simulink model "H250Model2019b"  (R2019b)
settings: Solver=ode4  StartTime=0.0  StopTime=inf  FixedStep=Ts  RelTol=1e-3
values from neighbouring files (symbols this model uses):
  ModelFail_env_P_wind = [0 0 0]    [F450DegradedParamInit.m]    (also in H250DegradedParamInit.m; H250ModelParam4S.m; H333DegradedParamInit4S.m)
  ModelFail_motor_isEnable = 0    [F450DegradedParamInit.m]    (also in H250DegradedParamInit.m; H250ModelParam4S.m; H333DegradedParamInit4S.m)
  ModelFail_motor_kCt = [1 1 1 1 1 1 1 1]    [F450DegradedParamInit.m]    (also in H250DegradedParamInit.m; H250ModelParam4S.m; H333DegradedParamInit4S.m)
  ModelFail_motor_kTc = [1 1 1 1 1 1 1 1]    [F450DegradedParamInit.m]    (also in H250DegradedParamInit.m; H250ModelParam4S.m; H333DegradedParamInit4S.m)
  ModelFail_motor_kw = [1 1 1 1 1 1 1 1]    [F450DegradedParamInit.m]    (also in H250DegradedParamInit.m; H250ModelParam4S.m; H333DegradedParamInit4S.m)
  ModelInit_motorInitRate = 0    [F450DegradedParamInit.m]    (also in H250DegradedParamInit.m; H250ModelParam4S.m; H333DegradedParamInit4S.m)
  ModelParam_Airframe_CMP = [0 0 0]    [F450DegradedParamInit.m]    (also in H250DegradedParamInit.m; H250ModelParam4S.m; H333DegradedParamInit4S.m)
  ModelParam_Airframe_J = [0.0194 0 0;0 0.0194 0;0 0 0.0291]    [F450DegradedParamInit.m]    (also in H250DegradedParamInit.m = [0.0056 0 0;0 0.0056 0;0 0 0.0104]; H250ModelParam4S.m = [0.0056 0 0;0 0.0056 0;0 0 0.0104]; H333DegradedParamInit4S.m = [0.012 0 0;0 0.012 0;0 0 0.02])
  ModelParam_Airframe_m = 1.31    [F450DegradedParamInit.m]    (also in H250DegradedParamInit.m = 0.752; H250ModelParam4S.m = 0.752; H333DegradedParamInit4S.m = 1.13)
  ModelParam_envAltitude = 0    [F450DegradedParamInit.m]    (also in H250DegradedParamInit.m; H250ModelParam4S.m; H333DegradedParamInit4S.m)
  ModelParam_envC_d = 0.055    [F450DegradedParamInit.m]    (also in H250DegradedParamInit.m; H250ModelParam4S.m; H333DegradedParamInit4S.m)
  ModelParam_envC_md = [0.001 0.001 0.00058]    [F450DegradedParamInit.m]    (also in H250DegradedParamInit.m = [0.001 0.001 0.00040]; H250ModelParam4S.m = [0.001 0.001 0.00040]; H333DegradedParamInit4S.m = [0.001 0.001 0.0002])
  ModelParam_GPSEphFinal = 0.3    [F450DegradedParamInit.m]    (also in H250DegradedParamInit.m; H250ModelParam4S.m; H333DegradedParamInit4S.m)
  ModelParam_GPSEpvFinal = 0.4    [F450DegradedParamInit.m]    (also in H250DegradedParamInit.m; H250ModelParam4S.m; H333DegradedParamInit4S.m)
  ModelParam_GPSFix3DFix = 3    [F450DegradedParamInit.m]    (also in H250DegradedParamInit.m; H250ModelParam4S.m; H333DegradedParamInit4S.m)
  ModelParam_GPSSatsVisible = 10    [F450DegradedParamInit.m]    (also in H250DegradedParamInit.m; H250ModelParam4S.m; H333DegradedParamInit4S.m)
  ModelParam_motorCr = 842.1    [F450DegradedParamInit.m]    (also in H250DegradedParamInit.m = 0; H250ModelParam4S.m = 0; H333DegradedParamInit4S.m = 0)
  ModelParam_motorFitType = 1    [F450DegradedParamInit.m]    (also in H250DegradedParamInit.m = 2; H250ModelParam4S.m = 2; H333DegradedParamInit4S.m = 2)
  ModelParam_motorJm = 0.0000687    (= 6.87e-05)    [F450DegradedParamInit.m]    (also in H250DegradedParamInit.m = 8.8493e-06; H250ModelParam4S.m = 8.8493e-06; H333DegradedParamInit4S.m = 8.8493e-06)
  ModelParam_motorMinThr = 0.05    [F450DegradedParamInit.m]    (also in H250DegradedParamInit.m = 0.148; H250ModelParam4S.m = 0.148; H333DegradedParamInit4S.m = 0.11)
  ModelParam_motorRateCurveCoeffi = [0 0 0]    [F450DegradedParamInit.m]    (also in H250DegradedParamInit.m = [-1364 3870 -372.4]; H250ModelParam4S.m = [-2143 5113 -458.4]; H333DegradedParamInit4S.m = [-1057 2662 -94.98])
  ModelParam_motorTc = 0.0214    [F450DegradedParamInit.m]    (also in H250DegradedParamInit.m = 0.035; H250ModelParam4S.m = 0.032; H333DegradedParamInit4S.m = 0.035)
  ModelParam_motorWb = 0    [F450DegradedParamInit.m]    (also in H250DegradedParamInit.m; H250ModelParam4S.m; H333DegradedParamInit4S.m)
  ModelParam_NoiseVarAcc0 = [0.1 0.1 0.1]    [F450DegradedParamInit.m]    (also in H250DegradedParamInit.m; H250ModelParam4S.m = [0.01 0.01 0.01]; H333DegradedParamInit4S.m)
  ModelParam_NoiseVarAcc1 = [0.1 0.1 0.1]    [F450DegradedParamInit.m]    (also in H250DegradedParamInit.m; H250ModelParam4S.m = [0.01 0.01 0.01]; H333DegradedParamInit4S.m)
  ModelParam_NoiseVarGPS_P0 = [1e-5 1e-5 1e-5]    [F450DegradedParamInit.m]    (also in H250DegradedParamInit.m; H250ModelParam4S.m; H333DegradedParamInit4S.m)
  ModelParam_NoiseVarGPS_V0 = [1e-5 1e-5 1e-5]    [F450DegradedParamInit.m]    (also in H250DegradedParamInit.m; H250ModelParam4S.m; H333DegradedParamInit4S.m)
  ModelParam_NoiseVarGyro0 = [0.0005 0.0005 0.0005]    [F450DegradedParamInit.m]    (also in H250DegradedParamInit.m; H250ModelParam4S.m; H333DegradedParamInit4S.m)
  ModelParam_NoiseVarGyro1 = [0.004 0.004 0.004]    [F450DegradedParamInit.m]    (also in H250DegradedParamInit.m; H250ModelParam4S.m; H333DegradedParamInit4S.m)
  ModelParam_NoiseVarMag0 = [0.000002 0.000002 0.000002]    [F450DegradedParamInit.m]    (also in H250DegradedParamInit.m; H250ModelParam4S.m; H333DegradedParamInit4S.m)
  ModelParam_NoiseVarMag1 = [0.0001 0.0001 0.0001]    [F450DegradedParamInit.m]    (also in H250DegradedParamInit.m; H250ModelParam4S.m; H333DegradedParamInit4S.m)
  ModelParam_PositionAcc0 = [0.071  0  -0.1365]    [F450DegradedParamInit.m]    (also in H250DegradedParamInit.m; H250ModelParam4S.m; H333DegradedParamInit4S.m)
  ModelParam_PositionAcc1 = [0.071  0  -0.1365]    [F450DegradedParamInit.m]    (also in H250DegradedParamInit.m; H250ModelParam4S.m; H333DegradedParamInit4S.m)
  ModelParam_rotorCt = 1.681e-05    [F450DegradedParamInit.m]    (also in H250DegradedParamInit.m = 1.448e-06; H250ModelParam4S.m = 1.345e-06; H333DegradedParamInit4S.m = 7.586e-06)
  ModelParam_WalkNoiseVarAcc0 = [0.001 0.001 0.001]    [F450DegradedParamInit.m]    (also in H250DegradedParamInit.m; H250ModelParam4S.m; H333DegradedParamInit4S.m)
  ModelParam_WalkNoiseVarAcc1 = [0.001 0.001 0.001]    [F450DegradedParamInit.m]    (also in H250DegradedParamInit.m; H250ModelParam4S.m; H333DegradedParamInit4S.m)
  ModelParam_WalkNoiseVarGPS_P0 = [0.01 0.01 0.01]    [F450DegradedParamInit.m]    (also in H250DegradedParamInit.m; H250ModelParam4S.m = [0 0 0]; H333DegradedParamInit4S.m)
  ModelParam_WalkNoiseVarGPS_V0 = [0.01 0.01 0.01]    [F450DegradedParamInit.m]    (also in H250DegradedParamInit.m; H250ModelParam4S.m = [0 0 0]; H333DegradedParamInit4S.m)
  ModelParam_WalkNoiseVarGyro0 = [0.00004 0.00004 0.00004]    [F450DegradedParamInit.m]    (also in H250DegradedParamInit.m; H250ModelParam4S.m; H333DegradedParamInit4S.m)
  ModelParam_WalkNoiseVarGyro1 = [0.00004 0.00004 0.00004]    [F450DegradedParamInit.m]    (also in H250DegradedParamInit.m; H250ModelParam4S.m; H333DegradedParamInit4S.m)
  ModelParam_WalkNoiseVarMag0 = [0.000001 0.000001 0.000001]    [F450DegradedParamInit.m]    (also in H250DegradedParamInit.m; H250ModelParam4S.m; H333DegradedParamInit4S.m)
  ModelParam_WalkNoiseVarMag1 = [0.000001 0.000001 0.000001]    [F450DegradedParamInit.m]    (also in H250DegradedParamInit.m; H250ModelParam4S.m; H333DegradedParamInit4S.m)
  MulticopterLayoutConfig = 1    [F450DegradedParamInit.m]    (also in H250DegradedParamInit.m = 6; H250ModelParam4S.m = 7; H333DegradedParamInit4S.m = 8)
  RflySimDisplayUAVType = 3    [F450DegradedParamInit.m]    (also in H250DegradedParamInit.m; H250ModelParam4S.m; H333DegradedParamInit4S.m)
  Ts = 1/1000    (= 0.001)    [F450DegradedParamInit.m]    (also in H250DegradedParamInit.m; H250ModelParam4S.m; H333DegradedParamInit4S.m)
undefined symbols (not defined in the file or in its folder): Earth, WGS84
libraries: aerolibnav x5, aerolibtransform2 x3, sharedtransform x3, aerolibutil x2, sharedutil x1, shared6dof x1, aerolibasang x1, aerolibatmos2 x1, aerolibconvert2 x1
(part 1 of 3)
settings Model: Creator=Jinrui  LastModifiedBy=kcx06
settings OptimizationCC: EfficientTunableParamExpr=on
settings DebuggingCC: ParameterTunabilityLossMsg=error  ArithmeticOperatorsInVariantConditions=warning
settings SFSimCC: SimUseLocalCustomCode=off  MATLABDynamicMemAlloc=off  CustomCodeUndefinedFunction=UseInterfaceOnly
settings RTWCC: SystemTargetFile=ert.tlc  GenCodeOnly=on  GenerateMakefile=off  PackageGeneratedCodeAndArtifacts=on  PackageName=MulticopterModel  TemplateMakefile=ert_default_tmf  RTWUseLocalCustomCode=off  TargetLang=C++  RTWCompilerOptimization=on
settings CodeAppCC: ForceParamTrailComments=on  OperatorAnnotations=on  SimulinkDataObjDesc=on  SFDataObjDesc=on  MATLABFcnDesc=on  InsertBlockDesc=on  StateflowObjectComments=on  MATLABSourceComments=on
settings ERTTargetCC: TargetLangStandard=C++03 (ISO)  MultiwordLength=2048  GenerateSampleERTMain=on  CodeInterfacePackaging=C++ class  SupportContinuousTime=on  SupportVariableSizeSignals=on  MultiInstanceErrorCode=None  RootIOFormat=Structure reference  ERTCustomFileTemplate=example_file_process.tlc  ERTFilePackagingFormat=Compact
settings SimscapeCC: SimscapeNormalizeSystem=off

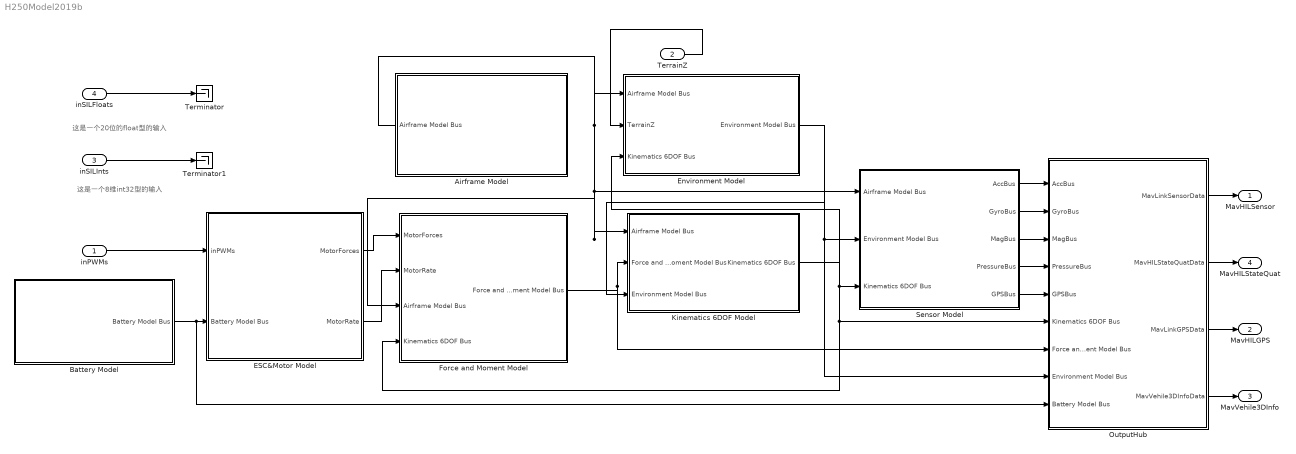
== system H250Model2019b ==
  note: 这是一个20位的float型的输入
  note: 这是一个8维int32型的输入
  inPWMs : Inport  PortDimensions=8
      settings: AttributesFormatString=Normalized PWM input with a range of [0-1]
  TerrainZ : Inport  Port=2  PortDimensions=1
  inSILInts : Inport  Port=3  OutDataTypeStr=int32  PortDimensions=8
  inSILFloats : Inport  Port=4  OutDataTypeStr=single  PortDimensions=20
  Airframe Model : Subsystem
  Battery Model : Subsystem
  ESC&Motor Model : Subsystem
  Environment Model : Subsystem
  Force and Moment Model : Subsystem
  Kinematics 6DOF Model : Subsystem
  OutputHub : Subsystem
  Sensor Model : Subsystem
  Terminator : Terminator
  Terminator1 : Terminator
  MavHILSensor : Outport  OutDataTypeStr=Bus: MavLinkSensor
  MavHILGPS : Outport  Port=2  OutDataTypeStr=Bus: MavLinkGPS
  MavVehile3DInfo : Outport  Port=3  OutDataTypeStr=Bus: MavVehileInfo
  MavHILStateQuat : Outport  Port=4  OutDataTypeStr=Bus: MavLinkStateQuat
  wires:
  Force and Moment Model/1(Force and Moment Model Bus) -> OutputHub/7(Force and Moment Model Bus), Kinematics 6DOF Model/2(Force and Moment Model Bus)
  inPWMs/1 -> ESC&Motor Model/1(inPWMs)
  ESC&Motor Model/1(MotorForces) -> Force and Moment Model/1(MotorForces)
  Sensor Model/5(GPSBus) -> OutputHub/5(GPSBus)
  Airframe Model/1(Airframe Model Bus) -> Kinematics 6DOF Model/1(Airframe Model Bus), Force and Moment Model/3(Airframe Model Bus), Sensor Model/1(Airframe Model Bus), Environment Model/1(Airframe Model Bus)
  Sensor Model/4(PressureBus) -> OutputHub/4(PressureBus)
  Sensor Model/2(GyroBus) -> OutputHub/2(GyroBus)
  OutputHub/4(MavVehile3DInfoData) -> MavVehile3DInfo/1
  OutputHub/3(MavLinkGPSData) -> MavHILGPS/1
  Environment Model/1(Environment Model Bus) -> Sensor Model/2(Environment Model Bus), OutputHub/8(Environment Model Bus), Kinematics 6DOF Model/3(Environment Model Bus)
  OutputHub/1(MavLinkSensorData) -> MavHILSensor/1
  Sensor Model/3(MagBus) -> OutputHub/3(MagBus)
  Sensor Model/1(AccBus) -> OutputHub/1(AccBus)
  Battery Model/1(Battery Model Bus) -> OutputHub/9(Battery Model Bus), ESC&Motor Model/2(Battery Model Bus)
  Kinematics 6DOF Model/1(Kinematics 6DOF Bus) -> Environment Model/3(Kinematics 6DOF Bus), Sensor Model/3(Kinematics 6DOF Bus), Force and Moment Model/4(Kinematics 6DOF Bus), OutputHub/6(Kinematics 6DOF Bus)
  ESC&Motor Model/2(MotorRate) -> Force and Moment Model/2(MotorRate)
  TerrainZ/1 -> Environment Model/2(TerrainZ)
  inSILInts/1 -> Terminator1/1
  inSILFloats/1 -> Terminator/1
  OutputHub/2(MavHILStateQuatData) -> MavHILStateQuat/1

== system H250Model2019b/Airframe Model ==
  ModelParam_Airframe_CenterOfMassPosition : Constant  Value=ModelParam_Airframe_CMP
  ModelParam_Airframe_J : Constant  Value=ModelParam_Airframe_J
  ModelParam_Airframe_m : Constant  Value=ModelParam_Airframe_m
  Out Bus Element1 : Outport  PortName=Airframe Model Bus  Element=m
  Out Bus Element2 : Outport  PortName=Airframe Model Bus  Element=J
  Out Bus Element : Outport  PortName=Airframe Model Bus  Element=CMP
  wires:
  ModelParam_Airframe_m/1 -> Out Bus Element1/1  "m_rt"
  ModelParam_Airframe_J/1 -> Out Bus Element2/1  "J_rt"
  ModelParam_Airframe_CenterOfMassPosition/1 -> Out Bus Element/1  "CMP_rt"

== system H250Model2019b/Battery Model ==
  BatteryVol : Constant  Value=12.6
  BatteryVolInit : Constant  Value=12.6
  Constant : Constant
  Constant1 : Constant
  Divide : Product  Inputs=*/
  Out Bus Element : Outport  PortName=Battery Model Bus  Element=BatteryEfficiency
  Out Bus Element1 : Outport  PortName=Battery Model Bus  Element=BattCellVoltage
  Out Bus Element2 : Outport  PortName=Battery Model Bus  Element=BattRemCapacity
  wires:
  BatteryVolInit/1 -> Divide/2
  BatteryVol/1 -> Divide/1
  Divide/1 -> Out Bus Element/1
  Constant/1 -> Out Bus Element1/1
  Constant1/1 -> Out Bus Element2/1

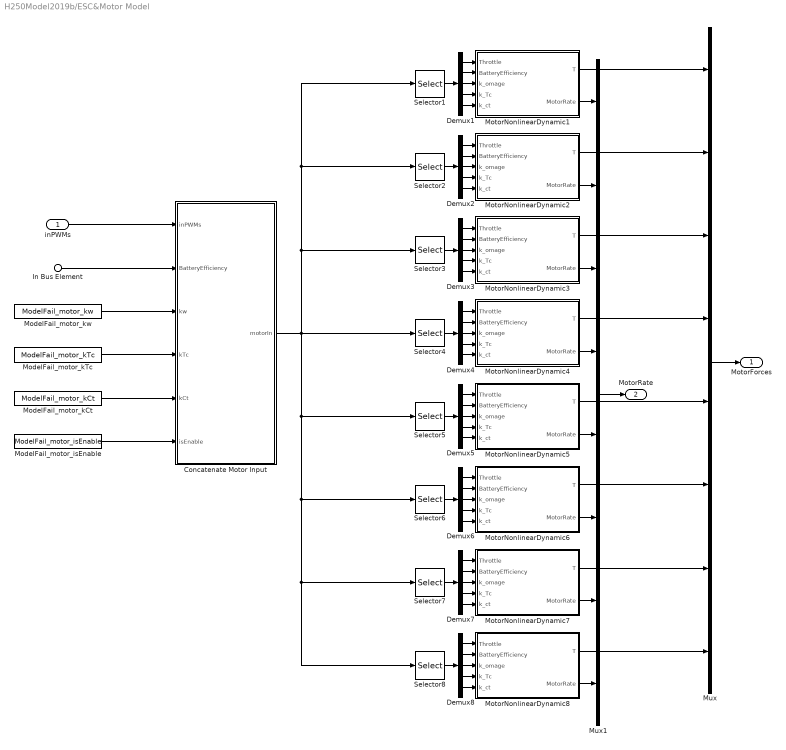
== system H250Model2019b/ESC&Motor Model ==
  inPWMs : Inport  PortDimensions=8
      settings: AttributesFormatString=Normalized PWM input with a range of [0-1]
  In Bus Element : Inport  Port=2  PortName=Battery Model Bus  Element=BatteryEfficiency
  Concatenate Motor Input : MATLAB Function  TreatAsAtomicUnit=on
  Demux{1..8} (8 alike) : Demux  Outputs=5
  ModelFail_motor_isEnable : Constant  Value=ModelFail_motor_isEnable
  ModelFail_motor_kCt : Constant  Value=ModelFail_motor_kCt
  ModelFail_motor_kTc : Constant  Value=ModelFail_motor_kTc
  ModelFail_motor_kw : Constant  Value=ModelFail_motor_kw
  MotorNonlinearDynamic1 : Subsystem  mask(ESC and Motor Model Block for Multicopter){motorInitRate=ModelInit_motorInitRate, motorFitType=ModelParam_motorFitType, motorCr=ModelParam_motorCr, motorWb=ModelParam_motorWb, motorRateCurveCoeffi=ModelParam_motorRateCurveCoeffi, motorTc=ModelParam_motorTc, rotorCt=ModelParam_rotorCt, MotorMinThr=ModelParam_motorMinThr}
      mask prompts: motorInitRate "Motor Initial Speed(rad/s)"; motorFitType "Motor_FitType"; motorCr "Motor_Cr"; motorWb "Motor_Wb"; motorRateCurveCoeffi "Motor_RateCurveCoeffi"; motorTc "Motor_Tc"; rotorCt "Rotor_Ct"; MotorMinThr "Dead Zone Throttle"
      mask TypeOptions motorInitRate: ModelInit_motorInitRate/Value
      mask TypeOptions motorFitType: ModelParam_motorFitType/Value
      mask TypeOptions motorCr: ModelParam_motorCr/Value
      mask TypeOptions motorWb: ModelParam_motorWb/Value
      mask TypeOptions motorRateCurveCoeffi: ModelParam_motorRateCurveCoeffi/Value
      mask TypeOptions motorTc: ModelParam_motorTc/Value
      mask TypeOptions rotorCt: ModelParam_rotorCt/Value
      mask TypeOptions MotorMinThr: ESC_MotorSteadyState/MotorMinThr
      mask DialogControl InitParam Prompt: Initial parameters
      mask DialogControl Param Prompt: Motor parameters
      mask Display:
      | port_label('input',1,'\sigma(0~1)','texmode','on');
      | port_label('input',2,'BatteryEfficiency(0~1)','texmode','on');
      | port_label('input',3,'k_{\varpi}','texmode','on');
      | port_label('input',4,'k_{Tc}','texmode','on');
      | port_label('input',5,'k_{Ct}','texmode','on');
      | 
      | port_label('output',1,'T(N)','texmode','on');
      | port_label('output', 2, '\varpi(rad/s)', 'texmode', 'on');
  MotorNonlinearDynamic2 : Subsystem  mask(ESC and Motor Model Block for Multicopter){motorInitRate=ModelInit_motorInitRate, motorFitType=ModelParam_motorFitType, motorCr=ModelParam_motorCr, motorWb=ModelParam_motorWb, motorRateCurveCoeffi=ModelParam_motorRateCurveCoeffi, motorTc=ModelParam_motorTc, rotorCt=ModelParam_rotorCt, MotorMinThr=ModelParam_motorMinThr}
      mask prompts: motorInitRate "Motor Initial Speed(rad/s)"; motorFitType "Motor_FitType"; motorCr "Motor_Cr"; motorWb "Motor_Wb"; motorRateCurveCoeffi "Motor_RateCurveCoeffi"; motorTc "Motor_Tc"; rotorCt "Rotor_Ct"; MotorMinThr "Dead Zone Throttle"
      mask TypeOptions motorInitRate: ModelInit_motorInitRate/Value
      mask TypeOptions motorFitType: ModelParam_motorFitType/Value
      mask TypeOptions motorCr: ModelParam_motorCr/Value
      mask TypeOptions motorWb: ModelParam_motorWb/Value
      mask TypeOptions motorRateCurveCoeffi: ModelParam_motorRateCurveCoeffi/Value
      mask TypeOptions motorTc: ModelParam_motorTc/Value
      mask TypeOptions rotorCt: ModelParam_rotorCt/Value
      mask TypeOptions MotorMinThr: ESC_MotorSteadyState/MotorMinThr
      mask DialogControl InitParam Prompt: Initial parameters
      mask DialogControl Param Prompt: Motor parameters
      mask Display:
      | port_label('input',1,'\sigma(0~1)','texmode','on');
      | port_label('input',2,'BatteryEfficiency(0~1)','texmode','on');
      | port_label('input',3,'k_{\varpi}','texmode','on');
      | port_label('input',4,'k_{Tc}','texmode','on');
      | port_label('input',5,'k_{Ct}','texmode','on');
      | 
      | port_label('output',1,'T(N)','texmode','on');
      | port_label('output', 2, '\varpi(rad/s)', 'texmode', 'on');
  MotorNonlinearDynamic3 : Subsystem  mask(ESC and Motor Model Block for Multicopter){motorInitRate=ModelInit_motorInitRate, motorFitType=ModelParam_motorFitType, motorCr=ModelParam_motorCr, motorWb=ModelParam_motorWb, motorRateCurveCoeffi=ModelParam_motorRateCurveCoeffi, motorTc=ModelParam_motorTc, rotorCt=ModelParam_rotorCt, MotorMinThr=ModelParam_motorMinThr}
      mask prompts: motorInitRate "Motor Initial Speed(rad/s)"; motorFitType "Motor_FitType"; motorCr "Motor_Cr"; motorWb "Motor_Wb"; motorRateCurveCoeffi "Motor_RateCurveCoeffi"; motorTc "Motor_Tc"; rotorCt "Rotor_Ct"; MotorMinThr "Dead Zone Throttle"
      mask TypeOptions motorInitRate: ModelInit_motorInitRate/Value
      mask TypeOptions motorFitType: ModelParam_motorFitType/Value
      mask TypeOptions motorCr: ModelParam_motorCr/Value
      mask TypeOptions motorWb: ModelParam_motorWb/Value
      mask TypeOptions motorRateCurveCoeffi: ModelParam_motorRateCurveCoeffi/Value
      mask TypeOptions motorTc: ModelParam_motorTc/Value
      mask TypeOptions rotorCt: ModelParam_rotorCt/Value
      mask TypeOptions MotorMinThr: ESC_MotorSteadyState/MotorMinThr
      mask DialogControl InitParam Prompt: Initial parameters
      mask DialogControl Param Prompt: Motor parameters
      mask Display:
      | port_label('input',1,'\sigma(0~1)','texmode','on');
      | port_label('input',2,'BatteryEfficiency(0~1)','texmode','on');
      | port_label('input',3,'k_{\varpi}','texmode','on');
      | port_label('input',4,'k_{Tc}','texmode','on');
      | port_label('input',5,'k_{Ct}','texmode','on');
      | 
      | port_label('output',1,'T(N)','texmode','on');
      | port_label('output', 2, '\varpi(rad/s)', 'texmode', 'on');
  MotorNonlinearDynamic4 : Subsystem  mask(ESC and Motor Model Block for Multicopter){motorInitRate=ModelInit_motorInitRate, motorFitType=ModelParam_motorFitType, motorCr=ModelParam_motorCr, motorWb=ModelParam_motorWb, motorRateCurveCoeffi=ModelParam_motorRateCurveCoeffi, motorTc=ModelParam_motorTc, rotorCt=ModelParam_rotorCt, MotorMinThr=ModelParam_motorMinThr}
      mask prompts: motorInitRate "Motor Initial Speed(rad/s)"; motorFitType "Motor_FitType"; motorCr "Motor_Cr"; motorWb "Motor_Wb"; motorRateCurveCoeffi "Motor_RateCurveCoeffi"; motorTc "Motor_Tc"; rotorCt "Rotor_Ct"; MotorMinThr "Dead Zone Throttle"
      mask TypeOptions motorInitRate: ModelInit_motorInitRate/Value
      mask TypeOptions motorFitType: ModelParam_motorFitType/Value
      mask TypeOptions motorCr: ModelParam_motorCr/Value
      mask TypeOptions motorWb: ModelParam_motorWb/Value
      mask TypeOptions motorRateCurveCoeffi: ModelParam_motorRateCurveCoeffi/Value
      mask TypeOptions motorTc: ModelParam_motorTc/Value
      mask TypeOptions rotorCt: ModelParam_rotorCt/Value
      mask TypeOptions MotorMinThr: ESC_MotorSteadyState/MotorMinThr
      mask DialogControl InitParam Prompt: Initial parameters
      mask DialogControl Param Prompt: Motor parameters
      mask Display:
      | port_label('input',1,'\sigma(0~1)','texmode','on');
      | port_label('input',2,'BatteryEfficiency(0~1)','texmode','on');
      | port_label('input',3,'k_{\varpi}','texmode','on');
      | port_label('input',4,'k_{Tc}','texmode','on');
      | port_label('input',5,'k_{Ct}','texmode','on');
      | 
      | port_label('output',1,'T(N)','texmode','on');
      | port_label('output', 2, '\varpi(rad/s)', 'texmode', 'on');
  MotorNonlinearDynamic5 : Subsystem  mask(ESC and Motor Model Block for Multicopter){motorInitRate=ModelInit_motorInitRate, motorFitType=ModelParam_motorFitType, motorCr=ModelParam_motorCr, motorWb=ModelParam_motorWb, motorRateCurveCoeffi=ModelParam_motorRateCurveCoeffi, motorTc=ModelParam_motorTc, rotorCt=ModelParam_rotorCt, MotorMinThr=ModelParam_motorMinThr}
      mask prompts: motorInitRate "Motor Initial Speed(rad/s)"; motorFitType "Motor_FitType"; motorCr "Motor_Cr"; motorWb "Motor_Wb"; motorRateCurveCoeffi "Motor_RateCurveCoeffi"; motorTc "Motor_Tc"; rotorCt "Rotor_Ct"; MotorMinThr "Dead Zone Throttle"
      mask TypeOptions motorInitRate: ModelInit_motorInitRate/Value
      mask TypeOptions motorFitType: ModelParam_motorFitType/Value
      mask TypeOptions motorCr: ModelParam_motorCr/Value
      mask TypeOptions motorWb: ModelParam_motorWb/Value
      mask TypeOptions motorRateCurveCoeffi: ModelParam_motorRateCurveCoeffi/Value
      mask TypeOptions motorTc: ModelParam_motorTc/Value
      mask TypeOptions rotorCt: ModelParam_rotorCt/Value
      mask TypeOptions MotorMinThr: ESC_MotorSteadyState/MotorMinThr
      mask DialogControl InitParam Prompt: Initial parameters
      mask DialogControl Param Prompt: Motor parameters
      mask Display:
      | port_label('input',1,'\sigma(0~1)','texmode','on');
      | port_label('input',2,'BatteryEfficiency(0~1)','texmode','on');
      | port_label('input',3,'k_{\varpi}','texmode','on');
      | port_label('input',4,'k_{Tc}','texmode','on');
      | port_label('input',5,'k_{Ct}','texmode','on');
      | 
      | port_label('output',1,'T(N)','texmode','on');
      | port_label('output', 2, '\varpi(rad/s)', 'texmode', 'on');
  MotorNonlinearDynamic6 : Subsystem  mask(ESC and Motor Model Block for Multicopter){motorInitRate=ModelInit_motorInitRate, motorFitType=ModelParam_motorFitType, motorCr=ModelParam_motorCr, motorWb=ModelParam_motorWb, motorRateCurveCoeffi=ModelParam_motorRateCurveCoeffi, motorTc=ModelParam_motorTc, rotorCt=ModelParam_rotorCt, MotorMinThr=ModelParam_motorMinThr}
      mask prompts: motorInitRate "Motor Initial Speed(rad/s)"; motorFitType "Motor_FitType"; motorCr "Motor_Cr"; motorWb "Motor_Wb"; motorRateCurveCoeffi "Motor_RateCurveCoeffi"; motorTc "Motor_Tc"; rotorCt "Rotor_Ct"; MotorMinThr "Dead Zone Throttle"
      mask TypeOptions motorInitRate: ModelInit_motorInitRate/Value
      mask TypeOptions motorFitType: ModelParam_motorFitType/Value
      mask TypeOptions motorCr: ModelParam_motorCr/Value
      mask TypeOptions motorWb: ModelParam_motorWb/Value
      mask TypeOptions motorRateCurveCoeffi: ModelParam_motorRateCurveCoeffi/Value
      mask TypeOptions motorTc: ModelParam_motorTc/Value
      mask TypeOptions rotorCt: ModelParam_rotorCt/Value
      mask TypeOptions MotorMinThr: ESC_MotorSteadyState/MotorMinThr
      mask DialogControl InitParam Prompt: Initial parameters
      mask DialogControl Param Prompt: Motor parameters
      mask Display:
      | port_label('input',1,'\sigma(0~1)','texmode','on');
      | port_label('input',2,'BatteryEfficiency(0~1)','texmode','on');
      | port_label('input',3,'k_{\varpi}','texmode','on');
      | port_label('input',4,'k_{Tc}','texmode','on');
      | port_label('input',5,'k_{Ct}','texmode','on');
      | 
      | port_label('output',1,'T(N)','texmode','on');
      | port_label('output', 2, '\varpi(rad/s)', 'texmode', 'on');
  MotorNonlinearDynamic7 : Subsystem  mask(ESC and Motor Model Block for Multicopter){motorInitRate=ModelInit_motorInitRate, motorFitType=ModelParam_motorFitType, motorCr=ModelParam_motorCr, motorWb=ModelParam_motorWb, motorRateCurveCoeffi=ModelParam_motorRateCurveCoeffi, motorTc=ModelParam_motorTc, rotorCt=ModelParam_rotorCt, MotorMinThr=ModelParam_motorMinThr}
      mask prompts: motorInitRate "Motor Initial Speed(rad/s)"; motorFitType "Motor_FitType"; motorCr "Motor_Cr"; motorWb "Motor_Wb"; motorRateCurveCoeffi "Motor_RateCurveCoeffi"; motorTc "Motor_Tc"; rotorCt "Rotor_Ct"; MotorMinThr "Dead Zone Throttle"
      mask TypeOptions motorInitRate: ModelInit_motorInitRate/Value
      mask TypeOptions motorFitType: ModelParam_motorFitType/Value
      mask TypeOptions motorCr: ModelParam_motorCr/Value
      mask TypeOptions motorWb: ModelParam_motorWb/Value
      mask TypeOptions motorRateCurveCoeffi: ModelParam_motorRateCurveCoeffi/Value
      mask TypeOptions motorTc: ModelParam_motorTc/Value
      mask TypeOptions rotorCt: ModelParam_rotorCt/Value
      mask TypeOptions MotorMinThr: ESC_MotorSteadyState/MotorMinThr
      mask DialogControl InitParam Prompt: Initial parameters
      mask DialogControl Param Prompt: Motor parameters
      mask Display:
      | port_label('input',1,'\sigma(0~1)','texmode','on');
      | port_label('input',2,'BatteryEfficiency(0~1)','texmode','on');
      | port_label('input',3,'k_{\varpi}','texmode','on');
      | port_label('input',4,'k_{Tc}','texmode','on');
      | port_label('input',5,'k_{Ct}','texmode','on');
      | 
      | port_label('output',1,'T(N)','texmode','on');
      | port_label('output', 2, '\varpi(rad/s)', 'texmode', 'on');
  MotorNonlinearDynamic8 : Subsystem  mask(ESC and Motor Model Block for Multicopter){motorInitRate=ModelInit_motorInitRate, motorFitType=ModelParam_motorFitType, motorCr=ModelParam_motorCr, motorWb=ModelParam_motorWb, motorRateCurveCoeffi=ModelParam_motorRateCurveCoeffi, motorTc=ModelParam_motorTc, rotorCt=ModelParam_rotorCt, MotorMinThr=ModelParam_motorMinThr}
      mask prompts: motorInitRate "Motor Initial Speed(rad/s)"; motorFitType "Motor_FitType"; motorCr "Motor_Cr"; motorWb "Motor_Wb"; motorRateCurveCoeffi "Motor_RateCurveCoeffi"; motorTc "Motor_Tc"; rotorCt "Rotor_Ct"; MotorMinThr "Dead Zone Throttle"
      mask TypeOptions motorInitRate: ModelInit_motorInitRate/Value
      mask TypeOptions motorFitType: ModelParam_motorFitType/Value
      mask TypeOptions motorCr: ModelParam_motorCr/Value
      mask TypeOptions motorWb: ModelParam_motorWb/Value
      mask TypeOptions motorRateCurveCoeffi: ModelParam_motorRateCurveCoeffi/Value
      mask TypeOptions motorTc: ModelParam_motorTc/Value
      mask TypeOptions rotorCt: ModelParam_rotorCt/Value
      mask TypeOptions MotorMinThr: ESC_MotorSteadyState/MotorMinThr
      mask DialogControl InitParam Prompt: Initial parameters
      mask DialogControl Param Prompt: Motor parameters
      mask Display:
      | port_label('input',1,'\sigma(0~1)','texmode','on');
      | port_label('input',2,'BatteryEfficiency(0~1)','texmode','on');
      | port_label('input',3,'k_{\varpi}','texmode','on');
      | port_label('input',4,'k_{Tc}','texmode','on');
      | port_label('input',5,'k_{Ct}','texmode','on');
      | 
      | port_label('output',1,'T(N)','texmode','on');
      | port_label('output', 2, '\varpi(rad/s)', 'texmode', 'on');
  Mux : Mux  Inputs=8
  Mux1 : Mux  Inputs=8
  Selector1 : Selector  NumberOfDimensions=2  InputPortWidth=3  IndexOptions=Select all,Index vector (dialog)  Indices=[1 3],1  OutputSizes=1,1
  Selector2 : Selector  NumberOfDimensions=2  InputPortWidth=3  IndexOptions=Select all,Index vector (dialog)  Indices=[1 3],2  OutputSizes=1,1
  Selector3 : Selector  NumberOfDimensions=2  InputPortWidth=3  IndexOptions=Select all,Index vector (dialog)  Indices=[1 3],3  OutputSizes=1,1
  Selector4 : Selector  NumberOfDimensions=2  InputPortWidth=3  IndexOptions=Select all,Index vector (dialog)  Indices=[1 3],4  OutputSizes=1,1
  Selector5 : Selector  NumberOfDimensions=2  InputPortWidth=3  IndexOptions=Select all,Index vector (dialog)  Indices=[1 3],5  OutputSizes=1,1
  Selector6 : Selector  NumberOfDimensions=2  InputPortWidth=3  IndexOptions=Select all,Index vector (dialog)  Indices=[1 3],6  OutputSizes=1,1
  Selector7 : Selector  NumberOfDimensions=2  InputPortWidth=3  IndexOptions=Select all,Index vector (dialog)  Indices=[1 3],7  OutputSizes=1,1
  Selector8 : Selector  NumberOfDimensions=2  InputPortWidth=3  IndexOptions=Select all,Index vector (dialog)  Indices=[1 3],8  OutputSizes=1,1
  MotorForces : Outport
  MotorRate : Outport  Port=2
  wires:
  inPWMs/1 -> Concatenate Motor Input/1(inPWMs)
  MotorNonlinearDynamic8/1(T) -> Mux/8
  MotorNonlinearDynamic7/1(T) -> Mux/7
  MotorNonlinearDynamic6/1(T) -> Mux/6
  MotorNonlinearDynamic5/1(T) -> Mux/5
  MotorNonlinearDynamic4/1(T) -> Mux/4
  MotorNonlinearDynamic3/1(T) -> Mux/3
  MotorNonlinearDynamic2/1(T) -> Mux/2
  MotorNonlinearDynamic1/1(T) -> Mux/1
  Mux/1 -> MotorForces/1
  In Bus Element/1 -> Concatenate Motor Input/2(BatteryEfficiency)
  ModelFail_motor_kw/1 -> Concatenate Motor Input/3(kw)
  ModelFail_motor_kTc/1 -> Concatenate Motor Input/4(kTc)
  ModelFail_motor_kCt/1 -> Concatenate Motor Input/5(kCt)
  Concatenate Motor Input/1(motorIn) -> Selector8/1, Selector7/1, Selector6/1, Selector5/1, Selector4/1, Selector3/1, Selector2/1, Selector1/1
  Demux1/1 -> MotorNonlinearDynamic1/1(Throttle)
  Demux1/2 -> MotorNonlinearDynamic1/2(BatteryEfficiency)
  Demux1/3 -> MotorNonlinearDynamic1/3(k_omage)
  Demux1/4 -> MotorNonlinearDynamic1/4(k_Tc)
  Demux1/5 -> MotorNonlinearDynamic1/5(k_ct)
  Demux2/5 -> MotorNonlinearDynamic2/5(k_ct)
  Demux2/4 -> MotorNonlinearDynamic2/4(k_Tc)
  Demux2/3 -> MotorNonlinearDynamic2/3(k_omage)
  Demux2/2 -> MotorNonlinearDynamic2/2(BatteryEfficiency)
  Demux2/1 -> MotorNonlinearDynamic2/1(Throttle)
  Demux3/1 -> MotorNonlinearDynamic3/1(Throttle)
  Demux3/2 -> MotorNonlinearDynamic3/2(BatteryEfficiency)
  Demux3/3 -> MotorNonlinearDynamic3/3(k_omage)
  Demux3/4 -> MotorNonlinearDynamic3/4(k_Tc)
  Demux3/5 -> MotorNonlinearDynamic3/5(k_ct)
  Demux4/1 -> MotorNonlinearDynamic4/1(Throttle)
  Demux4/2 -> MotorNonlinearDynamic4/2(BatteryEfficiency)
  Demux4/3 -> MotorNonlinearDynamic4/3(k_omage)
  Demux4/4 -> MotorNonlinearDynamic4/4(k_Tc)
  Demux4/5 -> MotorNonlinearDynamic4/5(k_ct)
  Demux5/1 -> MotorNonlinearDynamic5/1(Throttle)
  Demux5/2 -> MotorNonlinearDynamic5/2(BatteryEfficiency)
  Demux5/3 -> MotorNonlinearDynamic5/3(k_omage)
  Demux5/4 -> MotorNonlinearDynamic5/4(k_Tc)
  Demux5/5 -> MotorNonlinearDynamic5/5(k_ct)
  Demux6/1 -> MotorNonlinearDynamic6/1(Throttle)
  Demux6/2 -> MotorNonlinearDynamic6/2(BatteryEfficiency)
  Demux6/3 -> MotorNonlinearDynamic6/3(k_omage)
  Demux6/4 -> MotorNonlinearDynamic6/4(k_Tc)
  Demux6/5 -> MotorNonlinearDynamic6/5(k_ct)
  Demux7/1 -> MotorNonlinearDynamic7/1(Throttle)
  Demux7/2 -> MotorNonlinearDynamic7/2(BatteryEfficiency)
  Demux7/3 -> MotorNonlinearDynamic7/3(k_omage)
  Demux7/4 -> MotorNonlinearDynamic7/4(k_Tc)
  Demux7/5 -> MotorNonlinearDynamic7/5(k_ct)
  Demux8/1 -> MotorNonlinearDynamic8/1(Throttle)
  Demux8/2 -> MotorNonlinearDynamic8/2(BatteryEfficiency)
  Demux8/3 -> MotorNonlinearDynamic8/3(k_omage)
  Demux8/4 -> MotorNonlinearDynamic8/4(k_Tc)
  Demux8/5 -> MotorNonlinearDynamic8/5(k_ct)
  Selector1/1 -> Demux1/1
  Selector2/1 -> Demux2/1
  Selector3/1 -> Demux3/1
  Selector4/1 -> Demux4/1
  Selector5/1 -> Demux5/1
  Selector6/1 -> Demux6/1
  Selector7/1 -> Demux7/1
  Selector8/1 -> Demux8/1
  ModelFail_motor_isEnable/1 -> Concatenate Motor Input/6(isEnable)
  MotorNonlinearDynamic1/2(MotorRate) -> Mux1/1
  MotorNonlinearDynamic2/2(MotorRate) -> Mux1/2
  MotorNonlinearDynamic3/2(MotorRate) -> Mux1/3
  MotorNonlinearDynamic4/2(MotorRate) -> Mux1/4
  MotorNonlinearDynamic5/2(MotorRate) -> Mux1/5
  MotorNonlinearDynamic6/2(MotorRate) -> Mux1/6
  MotorNonlinearDynamic7/2(MotorRate) -> Mux1/7
  MotorNonlinearDynamic8/2(MotorRate) -> Mux1/8
  Mux1/1 -> MotorRate/1

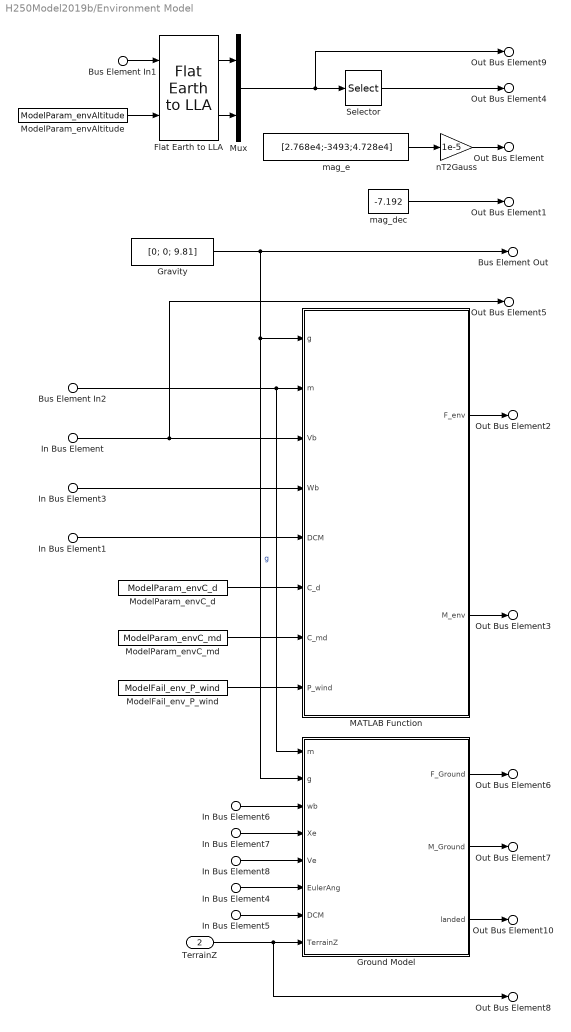
== system H250Model2019b/Environment Model ==
  Bus Element In2 : Inport  PortName=Airframe Model Bus  Element=m
  TerrainZ : Inport  Port=2
  Bus Element In1 : Inport  Port=3  PortName=Kinematics 6DOF Bus  Element=Xe
  In Bus Element7 : Inport  Port=3  PortName=Kinematics 6DOF Bus  Element=Xe
  In Bus Element : Inport  Port=3  PortName=Kinematics 6DOF Bus  Element=Vb
  In Bus Element1 : Inport  Port=3  PortName=Kinematics 6DOF Bus  Element=DCM
  In Bus Element5 : Inport  Port=3  PortName=Kinematics 6DOF Bus  Element=DCM
  In Bus Element3 : Inport  Port=3  PortName=Kinematics 6DOF Bus  Element=Wb
  In Bus Element6 : Inport  Port=3  PortName=Kinematics 6DOF Bus  Element=Wb
  In Bus Element4 : Inport  Port=3  PortName=Kinematics 6DOF Bus  Element=Euler
  In Bus Element8 : Inport  Port=3  PortName=Kinematics 6DOF Bus  Element=Ve
  Flat Earth to LLA : aerolibtransform2/Flat Earth to LLA  units=Metric (MKS)  ptype=Earth (WGS84)  F=1/298.257223563  R=6378137  LL0=ModelParam_GPSLatLong  psi=0
  Gravity : Constant  Value=[0; 0; 9.81]
  Ground Model : Subsystem
  MATLAB Function : MATLAB Function  TreatAsAtomicUnit=on
  ModelFail_env_P_wind : Constant  Value=ModelFail_env_P_wind
  ModelParam_envAltitude : Constant  Value=ModelParam_envAltitude
  ModelParam_envC_d : Constant  Value=ModelParam_envC_d
  ModelParam_envC_md : Constant  Value=ModelParam_envC_md
  Mux : Mux  Inputs=2
  Selector : Selector  InputPortWidth=3  IndexOptions=Index vector (dialog)  Indices=3  OutputSizes=1
  mag_dec : Constant  Value=-7.192
  mag_e : Constant  Value=[2.768e4;-3493;4.728e4]
  nT2Gauss : Gain  Gain=1e-5
  Bus Element Out : Outport  PortName=Environment Model Bus  Element=g
  Out Bus Element : Outport  PortName=Environment Model Bus  Element=mag_e
  Out Bus Element1 : Outport  PortName=Environment Model Bus  Element=mag_dec
  Out Bus Element2 : Outport  PortName=Environment Model Bus  Element=F_env
  Out Bus Element3 : Outport  PortName=Environment Model Bus  Element=M_env
  Out Bus Element4 : Outport  PortName=Environment Model Bus  Element=Altitude
  Out Bus Element6 : Outport  PortName=Environment Model Bus  Element=F_Ground
  Out Bus Element7 : Outport  PortName=Environment Model Bus  Element=M_Ground
  Out Bus Element8 : Outport  PortName=Environment Model Bus  Element=TerrainZ
  Out Bus Element9 : Outport  PortName=Environment Model Bus  Element=PosGPS
  Out Bus Element10 : Outport  PortName=Environment Model Bus  Element=landed
  Out Bus Element5 : Outport  PortName=Environment Model Bus  Element=V_wind_b_relative
  wires:
  Bus Element In1/1 -> Flat Earth to LLA/1
  ModelParam_envAltitude/1 -> Flat Earth to LLA/2
  Flat Earth to LLA/1 -> Mux/1
  Flat Earth to LLA/2 -> Mux/2
  Mux/1 -> Selector/1, Out Bus Element9/1
  Gravity/1 -> Bus Element Out/1, Ground Model/2(g), MATLAB Function/1(g)  "g"
  Selector/1 -> Out Bus Element4/1
  mag_e/1 -> nT2Gauss/1
  mag_dec/1 -> Out Bus Element1/1
  nT2Gauss/1 -> Out Bus Element/1
  In Bus Element/1 -> Out Bus Element5/1, MATLAB Function/3(Vb)
  In Bus Element1/1 -> MATLAB Function/5(DCM)
  In Bus Element3/1 -> MATLAB Function/4(Wb)
  MATLAB Function/2(M_env) -> Out Bus Element3/1
  MATLAB Function/1(F_env) -> Out Bus Element2/1
  ModelParam_envC_d/1 -> MATLAB Function/6(C_d)
  ModelParam_envC_md/1 -> MATLAB Function/7(C_md)
  ModelFail_env_P_wind/1 -> MATLAB Function/8(P_wind)
  In Bus Element4/1 -> Ground Model/6(EulerAng)
  In Bus Element5/1 -> Ground Model/7(DCM)
  In Bus Element6/1 -> Ground Model/3(wb)
  In Bus Element8/1 -> Ground Model/5(Ve)
  Bus Element In2/1 -> MATLAB Function/2(m), Ground Model/1(m)
  TerrainZ/1 -> Out Bus Element8/1, Ground Model/8(TerrainZ)
  Ground Model/2(M_Ground) -> Out Bus Element7/1
  Ground Model/1(F_Ground) -> Out Bus Element6/1
  In Bus Element7/1 -> Ground Model/4(Xe)
  Ground Model/3(landed) -> Out Bus Element10/1

== system H250Model2019b/Force and Moment Model ==
  MotorForces : Inport
  MotorRate : Inport  Port=2
  In Bus Element1 : Inport  Port=3  PortName=Airframe Model Bus  Element=CMP
  In Bus Element : Inport  Port=4  PortName=Kinematics 6DOF Bus  Element=Wb
  Add1 : Sum
  Allocation Model : Subsystem
  Gain1 : Gain  Gain=60/2/pi
  MulticopterLayoutConfig : Constant  Value=MulticopterLayoutConfig
  Out Bus Element : Outport  PortName=Force and Moment Model Bus  Element=F_motor
  Out Bus Element1 : Outport  PortName=Force and Moment Model Bus  Element=M_motor
  Out Bus Element2 : Outport  PortName=Force and Moment Model Bus  Element=Motor_RPM
  wires:
  MulticopterLayoutConfig/1 -> Allocation Model/1(index)
  Allocation Model/1(F) -> Out Bus Element/1
  Allocation Model/2(M) -> Add1/1
  Allocation Model/3(M_G) -> Add1/2
  Add1/1 -> Out Bus Element1/1
  MotorForces/1 -> Allocation Model/2(MotorForces)
  Gain1/1 -> Out Bus Element2/1
  MotorRate/1 -> Gain1/1, Allocation Model/5(MotorRate)
  In Bus Element/1 -> Allocation Model/3(Wb)
  In Bus Element1/1 -> Allocation Model/4(o_m)

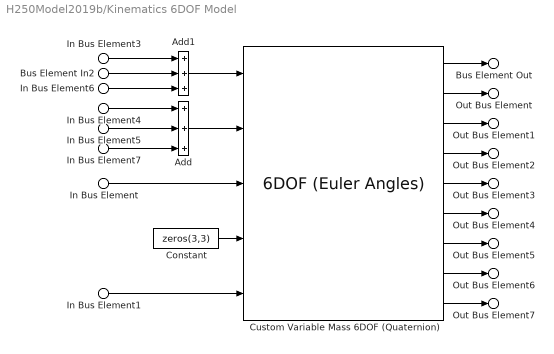
== system H250Model2019b/Kinematics 6DOF Model ==
  In Bus Element : Inport  PortName=Airframe Model Bus  Element=m
  In Bus Element1 : Inport  PortName=Airframe Model Bus  Element=J
  In Bus Element3 : Inport  Port=2  PortName=Force and Moment Model Bus  Element=F_motor
  In Bus Element4 : Inport  Port=2  PortName=Force and Moment Model Bus  Element=M_motor
  Bus Element In2 : Inport  Port=3  PortName=Environment Model Bus  Element=F_env
  In Bus Element5 : Inport  Port=3  PortName=Environment Model Bus  Element=M_env
  In Bus Element6 : Inport  Port=3  PortName=Environment Model Bus  Element=F_Ground
  In Bus Element7 : Inport  Port=3  PortName=Environment Model Bus  Element=M_Ground
  Add : Sum  Inputs=+++
  Add1 : Sum  Inputs=+++
  Constant : Constant  Value=zeros(3,3)
  Custom Variable Mass 6DOF (Quaternion) : shared6dof/6DOF (Euler Angles)  units=Metric (MKS)  mtype=Custom Variable  rep=Quaternion  xme_0=ModelInit_PosE  Vm_0=ModelInit_VelB  eul_0=ModelInit_AngEuler  pm_0=ModelInit_RateB  mass_0=1.0  mass_e=0.5  mass_f=2.0  inertia=eye(3)  inertia_e=eye(3)  inertia_f=2*eye(3)  k_quat=1.0  vre_flag=off  abi_flag=on  aMode=0  xme_statename=''  Vm_statename=''  eul_statename=''  quat_statename=''  pm_statename=''  mass_statename=''
      settings: SourceProductBaseCode=AE,PW,MT,UV,VE,VP
  Bus Element Out : Outport  PortName=Kinematics 6DOF Bus  Element=Ve
  Out Bus Element : Outport  PortName=Kinematics 6DOF Bus  Element=Xe
  Out Bus Element1 : Outport  PortName=Kinematics 6DOF Bus  Element=Euler
  Out Bus Element2 : Outport  PortName=Kinematics 6DOF Bus  Element=DCM
  Out Bus Element3 : Outport  PortName=Kinematics 6DOF Bus  Element=Vb
  Out Bus Element4 : Outport  PortName=Kinematics 6DOF Bus  Element=Wb
  Out Bus Element5 : Outport  PortName=Kinematics 6DOF Bus  Element=dWb
  Out Bus Element6 : Outport  PortName=Kinematics 6DOF Bus  Element=Abb
  Out Bus Element7 : Outport  PortName=Kinematics 6DOF Bus  Element=Abe
  wires:
  In Bus Element3/1 -> Add1/1
  In Bus Element4/1 -> Add/1
  In Bus Element/1 -> Custom Variable Mass 6DOF (Quaternion)/3
  Constant/1 -> Custom Variable Mass 6DOF (Quaternion)/4
  In Bus Element1/1 -> Custom Variable Mass 6DOF (Quaternion)/5
  Custom Variable Mass 6DOF (Quaternion)/1 -> Bus Element Out/1
  Custom Variable Mass 6DOF (Quaternion)/2 -> Out Bus Element/1
  Custom Variable Mass 6DOF (Quaternion)/9 -> Out Bus Element7/1
  Custom Variable Mass 6DOF (Quaternion)/8 -> Out Bus Element6/1
  Custom Variable Mass 6DOF (Quaternion)/7 -> Out Bus Element5/1
  Custom Variable Mass 6DOF (Quaternion)/6 -> Out Bus Element4/1
  Custom Variable Mass 6DOF (Quaternion)/5 -> Out Bus Element3/1
  Custom Variable Mass 6DOF (Quaternion)/4 -> Out Bus Element2/1
  Custom Variable Mass 6DOF (Quaternion)/3 -> Out Bus Element1/1
  Bus Element In2/1 -> Add1/2
  In Bus Element5/1 -> Add/2
  Add1/1 -> Custom Variable Mass 6DOF (Quaternion)/1
  Add/1 -> Custom Variable Mass 6DOF (Quaternion)/2
  In Bus Element6/1 -> Add1/3
  In Bus Element7/1 -> Add/3

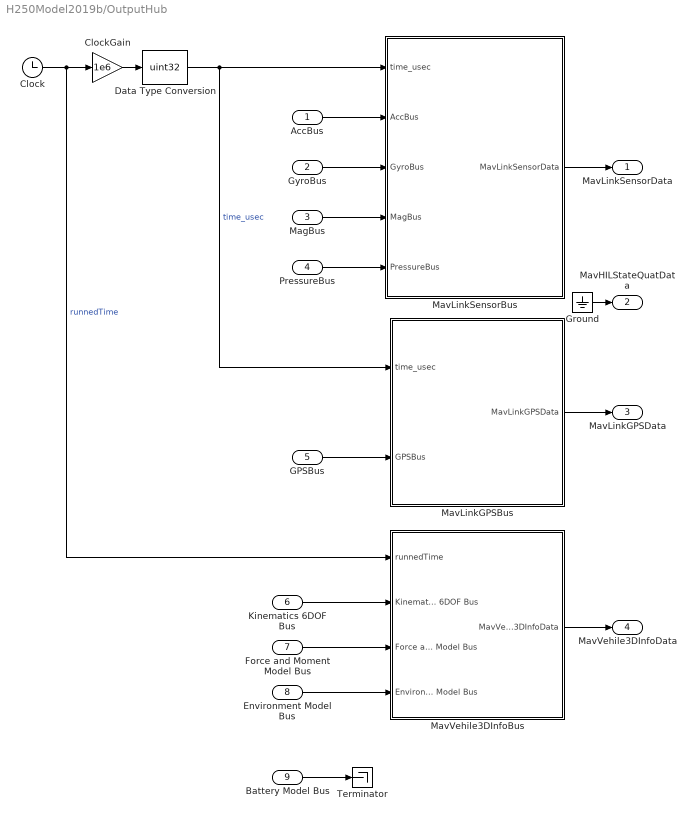
== system H250Model2019b/OutputHub ==
  AccBus : Inport
  GyroBus : Inport  Port=2
  MagBus : Inport  Port=3
  PressureBus : Inport  Port=4
  GPSBus : Inport  Port=5
  Kinematics 6DOF Bus : Inport  Port=6
  Force and Moment Model Bus : Inport  Port=7
  Environment Model Bus : Inport  Port=8
  Battery Model Bus : Inport  Port=9
  Clock : Clock
  ClockGain : Gain  Gain=1e6
  Data Type Conversion : DataTypeConversion  OutDataTypeStr=uint32
  Ground : Ground
  MavLinkGPSBus : Subsystem
  MavLinkSensorBus : Subsystem
  MavVehile3DInfoBus : Subsystem
  Terminator : Terminator
  MavLinkSensorData : Outport  OutDataTypeStr=Bus: MavLinkSensor
  MavHILStateQuatData : Outport  Port=2  OutDataTypeStr=Bus: MavLinkStateQuat
  MavLinkGPSData : Outport  Port=3  OutDataTypeStr=Bus: MavLinkGPS
  MavVehile3DInfoData : Outport  Port=4  OutDataTypeStr=Bus: MavVehileInfo
  wires:
  Clock/1 -> MavVehile3DInfoBus/1(runnedTime), ClockGain/1  "runnedTime"
  ClockGain/1 -> Data Type Conversion/1
  Data Type Conversion/1 -> MavLinkGPSBus/1(time_usec), MavLinkSensorBus/1(time_usec)  "time_usec"
  AccBus/1 -> MavLinkSensorBus/2(AccBus)
  GyroBus/1 -> MavLinkSensorBus/3(GyroBus)
  MagBus/1 -> MavLinkSensorBus/4(MagBus)
  PressureBus/1 -> MavLinkSensorBus/5(PressureBus)
  MavLinkSensorBus/1(MavLinkSensorData) -> MavLinkSensorData/1
  GPSBus/1 -> MavLinkGPSBus/2(GPSBus)
  MavLinkGPSBus/1(MavLinkGPSData) -> MavLinkGPSData/1
  MavVehile3DInfoBus/1(MavVehile3DInfoData) -> MavVehile3DInfoData/1
  Force and Moment Model Bus/1 -> MavVehile3DInfoBus/3(Force and Moment Model Bus)
  Kinematics 6DOF Bus/1 -> MavVehile3DInfoBus/2(Kinematics 6DOF Bus)
  Ground/1 -> MavHILStateQuatData/1
  Environment Model Bus/1 -> MavVehile3DInfoBus/4(Environment Model Bus)
  Battery Model Bus/1 -> Terminator/1

== system H250Model2019b/Sensor Model ==
  Airframe Model Bus : Inport
  Environment Model Bus : Inport  Port=2
  Kinematics 6DOF Bus : Inport  Port=3
  Acc Bus Creator : BusCreator  Inputs=2
  Accelerometer Hub : Subsystem
  Barometer : Subsystem
  GPS : Subsystem
  Gyro Bus Creator : BusCreator  Inputs=2
  Gyroscope Hub : Subsystem
  Mag Bus Creator : BusCreator  Inputs=2
  Magnetometer Hub : Subsystem
  Pressure Bus Creator : BusCreator  Inputs=3
  AccBus : Outport
  GyroBus : Outport  Port=2
  MagBus : Outport  Port=3
  PressureBus : Outport  Port=4
  GPSBus : Outport  Port=5
  wires:
  Environment Model Bus/1 -> Magnetometer Hub/2(Environment Model Bus), Barometer/1(Environment Model Bus), Accelerometer Hub/1(Environment Model Bus)
  Kinematics 6DOF Bus/1 -> Accelerometer Hub/2(Kinematics 6DOF Bus), GPS/1(Kinematics 6DOF Bus), Magnetometer Hub/1(Kinematics 6DOF Bus), Gyroscope Hub/1(Kinematics 6DOF Bus)
  Accelerometer Hub/1(Ameans0) -> Acc Bus Creator/1  "Ameans0"
  GPS/1(GPS) -> GPSBus/1
  Barometer/1(Pressure) -> Pressure Bus Creator/1  "Pressure_abs"
  Accelerometer Hub/2(Ameans1) -> Acc Bus Creator/2  "Ameans1"
  Acc Bus Creator/1 -> AccBus/1
  Gyroscope Hub/1(Wmeans0) -> Gyro Bus Creator/1  "Wmeans0"
  Gyroscope Hub/2(Wmeans1) -> Gyro Bus Creator/2  "Wmeans1"
  Magnetometer Hub/1(Mag_means0) -> Mag Bus Creator/1  "Mag_means0"
  Magnetometer Hub/2(Mag_means1) -> Mag Bus Creator/2  "Mag_means1"
  Gyro Bus Creator/1 -> GyroBus/1
  Mag Bus Creator/1 -> MagBus/1
  Pressure Bus Creator/1 -> PressureBus/1
  Barometer/2(PressureAlt) -> Pressure Bus Creator/2  "PressureAlt"
  Barometer/3(diff_pressure) -> Pressure Bus Creator/3  "Pressure_diff"
  Airframe Model Bus/1 -> Accelerometer Hub/3(Airframe Model Bus)

== system H250Model2019b/ESC&Motor Model/MotorNonlinearDynamic1 ==
  Throttle : Inport
  BatteryEfficiency : Inport  Port=2  Unit=V
  k_omage : Inport  Port=3
  k_Tc : Inport  Port=4
  k_ct : Inport  Port=5
  ESC_MotorSteadyState : MATLAB Function  TreatAsAtomicUnit=on  mask{MotorMinThr=MotorMinThr}
      mask prompts: MotorMinThr "Minimum Throttle"
  ModelInit_motorInitRate : Constant  Value=motorInitRate
  ModelParam_motorCr : Constant  Value=motorCr
  ModelParam_motorFitType : Constant  Value=motorFitType
  ModelParam_motorRateCurveCoeffi : Constant  Value=motorRateCurveCoeffi
  ModelParam_motorTc : Constant  Value=motorTc
  ModelParam_motorWb : Constant  Value=motorWb
  ModelParam_rotorCt : Constant  Value=rotorCt
  MotorDynamic : Subsystem
      mask Display:
      | port_label('input', 1, '\varpi_{ss}(rad/s)', 'texmode', 'on');
      | port_label('input', 2, '\varpi_{0}(rad/s)', 'texmode', 'on');
      | port_label('input', 3, 'T_{c}(s)', 'texmode', 'on');
      | port_label('output', 1, '\varpi(rad/s)', 'texmode', 'on');
  Product{,1..3} (4 alike) : Product
  Square : Math  Operator=square  SaturateOnIntegerOverflow=on
  T : Outport  Unit=N
  MotorRate : Outport  Port=2  Unit=rad/s
  wires:
  ModelParam_motorWb/1 -> ESC_MotorSteadyState/4(Ratebias)
  Throttle/1 -> ESC_MotorSteadyState/1(Throttle)
  ModelParam_motorCr/1 -> ESC_MotorSteadyState/3(Cr)
  ModelInit_motorInitRate/1 -> MotorDynamic/2(MotorInitRate)
  ModelParam_rotorCt/1 -> Product1/1
  Product/1 -> T/1
  ESC_MotorSteadyState/1(SteadyStateRate) -> Product3/2
  Square/1 -> Product/1
  ModelParam_motorTc/1 -> Product2/1
  MotorDynamic/1(MotorRate) -> MotorRate/1, Square/1
  BatteryEfficiency/1 -> ESC_MotorSteadyState/2(BatteryEfficiency)
  Product1/1 -> Product/2
  Product2/1 -> MotorDynamic/3(MotorTimeConstant)
  Product3/1 -> MotorDynamic/1(ReferenceRate)
  k_omage/1 -> Product3/1
  k_Tc/1 -> Product2/2
  k_ct/1 -> Product1/2
  ModelParam_motorRateCurveCoeffi/1 -> ESC_MotorSteadyState/5(MotorRateCurveCoeffi)
  ModelParam_motorFitType/1 -> ESC_MotorSteadyState/6(MotorFitType)

== system H250Model2019b/ESC&Motor Model/MotorNonlinearDynamic2 ==
  Throttle : Inport
  BatteryEfficiency : Inport  Port=2  Unit=V
  k_omage : Inport  Port=3
  k_Tc : Inport  Port=4
  k_ct : Inport  Port=5
  ESC_MotorSteadyState : MATLAB Function  TreatAsAtomicUnit=on  mask{MotorMinThr=MotorMinThr}
      mask prompts: MotorMinThr "Minimum Throttle"
  ModelInit_motorInitRate : Constant  Value=motorInitRate
  ModelParam_motorCr : Constant  Value=motorCr
  ModelParam_motorFitType : Constant  Value=motorFitType
  ModelParam_motorRateCurveCoeffi : Constant  Value=motorRateCurveCoeffi
  ModelParam_motorTc : Constant  Value=motorTc
  ModelParam_motorWb : Constant  Value=motorWb
  ModelParam_rotorCt : Constant  Value=rotorCt
  MotorDynamic : Subsystem
      mask Display:
      | port_label('input', 1, '\varpi_{ss}(rad/s)', 'texmode', 'on');
      | port_label('input', 2, '\varpi_{0}(rad/s)', 'texmode', 'on');
      | port_label('input', 3, 'T_{c}(s)', 'texmode', 'on');
      | port_label('output', 1, '\varpi(rad/s)', 'texmode', 'on');
  Product{,1..3} (4 alike) : Product
  Square : Math  Operator=square  SaturateOnIntegerOverflow=on
  T : Outport  Unit=N
  MotorRate : Outport  Port=2  Unit=rad/s
  wires:
  ModelParam_motorFitType/1 -> ESC_MotorSteadyState/6(MotorFitType)
  ModelParam_motorRateCurveCoeffi/1 -> ESC_MotorSteadyState/5(MotorRateCurveCoeffi)
  k_ct/1 -> Product1/2
  k_Tc/1 -> Product2/2
  k_omage/1 -> Product3/1
  Product3/1 -> MotorDynamic/1(ReferenceRate)
  Product2/1 -> MotorDynamic/3(MotorTimeConstant)
  Product1/1 -> Product/2
  BatteryEfficiency/1 -> ESC_MotorSteadyState/2(BatteryEfficiency)
  MotorDynamic/1(MotorRate) -> Square/1, MotorRate/1
  ModelParam_motorTc/1 -> Product2/1
  Square/1 -> Product/1
  ESC_MotorSteadyState/1(SteadyStateRate) -> Product3/2
  Product/1 -> T/1
  ModelParam_rotorCt/1 -> Product1/1
  ModelInit_motorInitRate/1 -> MotorDynamic/2(MotorInitRate)
  ModelParam_motorCr/1 -> ESC_MotorSteadyState/3(Cr)
  Throttle/1 -> ESC_MotorSteadyState/1(Throttle)
  ModelParam_motorWb/1 -> ESC_MotorSteadyState/4(Ratebias)

== system H250Model2019b/ESC&Motor Model/MotorNonlinearDynamic3 ==
  Throttle : Inport
  BatteryEfficiency : Inport  Port=2  Unit=V
  k_omage : Inport  Port=3
  k_Tc : Inport  Port=4
  k_ct : Inport  Port=5
  ESC_MotorSteadyState : MATLAB Function  TreatAsAtomicUnit=on  mask{MotorMinThr=MotorMinThr}
      mask prompts: MotorMinThr "Minimum Throttle"
  ModelInit_motorInitRate : Constant  Value=motorInitRate
  ModelParam_motorCr : Constant  Value=motorCr
  ModelParam_motorFitType : Constant  Value=motorFitType
  ModelParam_motorRateCurveCoeffi : Constant  Value=motorRateCurveCoeffi
  ModelParam_motorTc : Constant  Value=motorTc
  ModelParam_motorWb : Constant  Value=motorWb
  ModelParam_rotorCt : Constant  Value=rotorCt
  MotorDynamic : Subsystem
      mask Display:
      | port_label('input', 1, '\varpi_{ss}(rad/s)', 'texmode', 'on');
      | port_label('input', 2, '\varpi_{0}(rad/s)', 'texmode', 'on');
      | port_label('input', 3, 'T_{c}(s)', 'texmode', 'on');
      | port_label('output', 1, '\varpi(rad/s)', 'texmode', 'on');
  Product{,1..3} (4 alike) : Product
  Square : Math  Operator=square  SaturateOnIntegerOverflow=on
  T : Outport  Unit=N
  MotorRate : Outport  Port=2  Unit=rad/s
  wires:
  ModelParam_motorWb/1 -> ESC_MotorSteadyState/4(Ratebias)
  Throttle/1 -> ESC_MotorSteadyState/1(Throttle)
  ModelParam_motorCr/1 -> ESC_MotorSteadyState/3(Cr)
  ModelInit_motorInitRate/1 -> MotorDynamic/2(MotorInitRate)
  ModelParam_rotorCt/1 -> Product1/1
  Product/1 -> T/1
  ESC_MotorSteadyState/1(SteadyStateRate) -> Product3/2
  Square/1 -> Product/1
  ModelParam_motorTc/1 -> Product2/1
  MotorDynamic/1(MotorRate) -> MotorRate/1, Square/1
  BatteryEfficiency/1 -> ESC_MotorSteadyState/2(BatteryEfficiency)
  Product1/1 -> Product/2
  Product2/1 -> MotorDynamic/3(MotorTimeConstant)
  Product3/1 -> MotorDynamic/1(ReferenceRate)
  k_omage/1 -> Product3/1
  k_Tc/1 -> Product2/2
  k_ct/1 -> Product1/2
  ModelParam_motorRateCurveCoeffi/1 -> ESC_MotorSteadyState/5(MotorRateCurveCoeffi)
  ModelParam_motorFitType/1 -> ESC_MotorSteadyState/6(MotorFitType)
